simulink model "simulation"  (R2020b)
settings: Solver=VariableStepAuto  StartTime=0.0  StopTime=100.0  RelTol=1e-3
values from neighbouring files (symbols this model uses):
  a_phi1 = 2.879    [linear_aircraft_model_constants.m]
  a_phi2 = -0.65    [linear_aircraft_model_constants.m]
  d = deg2rad(1.5)    [linear_aircraft_model_constants.m]
  delta_a_max = delta_a_max    [linear_aircraft_model_constants.m]
  g = 9.81    [linear_aircraft_model_constants.m]
  k_d_phi = (2*zeta_phi*omega_n_phi - a_phi1)/(a_phi2)    [linear_aircraft_model_constants.m]
  k_i_chi = omega_n_chi^2*V_g/g    [linear_aircraft_model_constants.m]
  k_i_phi = 0    [linear_aircraft_model_constants.m]    (also in oppg2.m = k_i_min + i*res)
  k_p_chi = 2*zeta_chi*omega_n_chi*V_g/g    [linear_aircraft_model_constants.m]
  k_p_phi = delta_a_max/e_phi_max * sign(a_phi2)    [linear_aircraft_model_constants.m]
  V_g = 580/3.6    (= 161.111111111)    [linear_aircraft_model_constants.m]
settings Model: Creator=danie  LastModifiedBy=danie

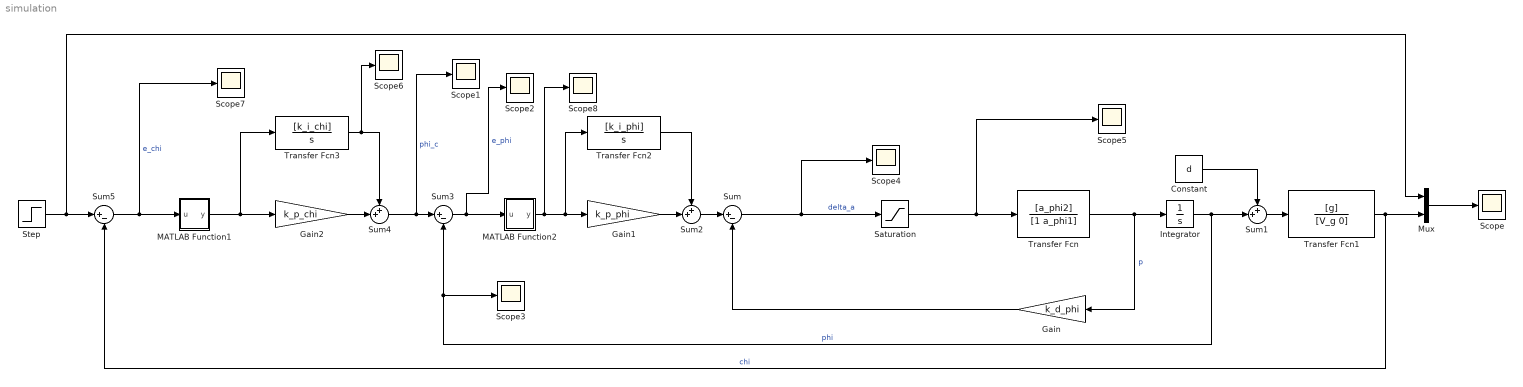
== system simulation ==
  Constant : Constant  Value=d
  Gain : Gain  Gain=k_d_phi
  Gain1 : Gain  Gain=k_p_phi
  Gain2 : Gain  Gain=k_p_chi
  Integrator : Integrator
  MATLAB Function1 : MATLAB Function  TreatAsAtomicUnit=on
  MATLAB Function2 : MATLAB Function  TreatAsAtomicUnit=on
  Mux : Mux  Inputs=2
  Saturation : Saturate  UpperLimit=delta_a_max  LowerLimit=-delta_a_max
  Scope{,1..8} (9 alike) : Scope
  Step : Step  Time=5  After=10*pi/180  SampleTime=0
  Sum : Sum  Inputs=|+-
  Sum1 : Sum  Inputs=++|
  Sum2 : Sum  Inputs=++|
  Sum3 : Sum  Inputs=|+-
  Sum4 : Sum  Inputs=++|
  Sum5 : Sum  Inputs=|+-
  Transfer Fcn : TransferFcn  Numerator=[a_phi2]  Denominator=[1 a_phi1]
  Transfer Fcn1 : TransferFcn  Numerator=[g]  Denominator=[V_g 0]
  Transfer Fcn2 : TransferFcn  Numerator=[k_i_phi]  Denominator=[1 0]
  Transfer Fcn3 : TransferFcn  Numerator=[k_i_chi]  Denominator=[1 0]
  wires:
  Sum/1 -> Saturation/1, Scope4/1  "delta_a"
  Transfer Fcn/1 -> Gain/1, Integrator/1  "p"
  Gain/1 -> Sum/2
  Integrator/1 -> Scope3/1, Sum3/2, Sum1/2  "phi"
  Constant/1 -> Sum1/1
  Sum1/1 -> Transfer Fcn1/1
  Transfer Fcn1/1 -> Mux/2, Sum5/2  "chi"
  Sum2/1 -> Sum/1
  Gain1/1 -> Sum2/2
  Transfer Fcn2/1 -> Sum2/1
  Sum3/1 -> MATLAB Function2/1(u), Scope2/1  "e_phi"
  Sum5/1 -> MATLAB Function1/1(u), Scope7/1  "e_chi"
  Transfer Fcn3/1 -> Scope6/1, Sum4/1
  Gain2/1 -> Sum4/2
  Sum4/1 -> Scope1/1, Sum3/1  "phi_c"
  Step/1 -> Mux/1, Sum5/1
  Mux/1 -> Scope/1
  Saturation/1 -> Scope5/1, Transfer Fcn/1
  MATLAB Function2/1(y) -> Scope8/1, Transfer Fcn2/1, Gain1/1
  MATLAB Function1/1(y) -> Transfer Fcn3/1, Gain2/1

== matlab function simulation/MATLAB Function2 ==
  data: u input; y output
function y = fcn(u)

y = angdiff(0,u);

== matlab function simulation/MATLAB Function1 ==
  data: u input; y output
function y = fcn(u)

y = angdiff(0,u);
